simulink model "deney42"  (R2023b)
settings: Solver=VariableStepAuto  StartTime=0.0  StopTime=20  RelTol=1e-3
libraries: commrandsrc3 x1, spsControlledVoltageSourceLib x1, spsDiodeLib x1, dspfdesign x1, spsParallelRLCBranchLib x1, spsVoltageMeasurementLib x1, sps_lib x1
settings Model: Creator=fatih  LastModifiedBy=fatih

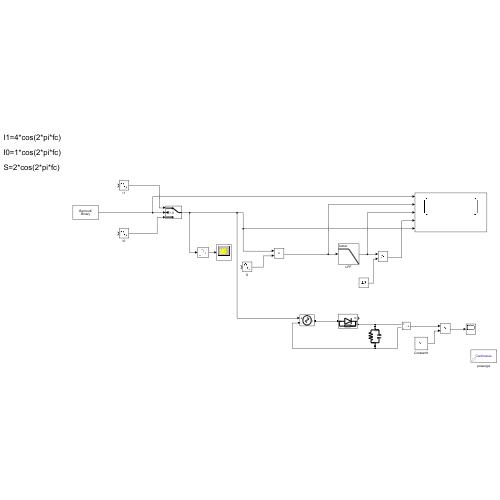
[thumbnail: Simulink's stored preview of the top-level diagram]
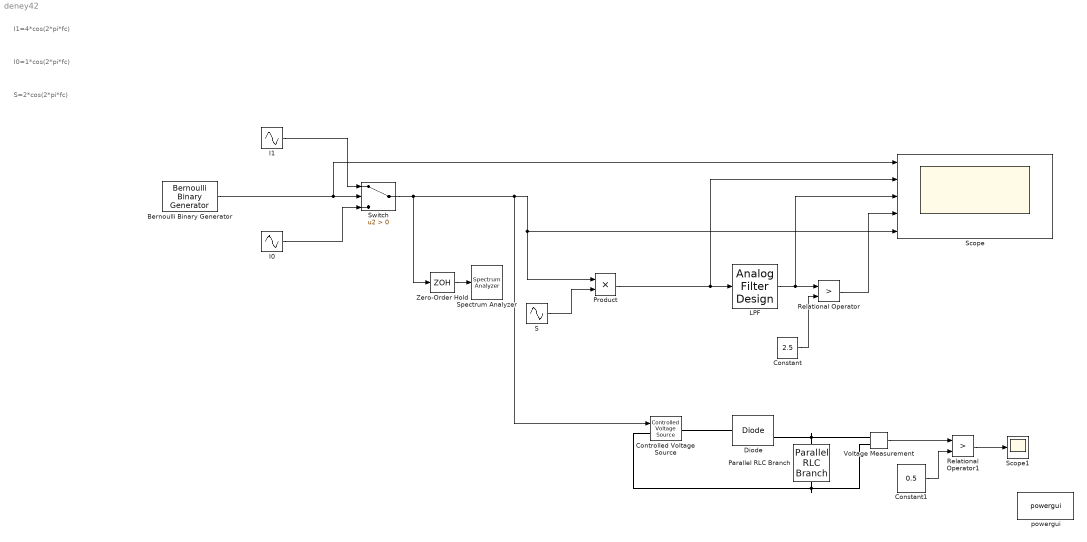
== system deney42 ==
  note: S=2*cos(2*pi*fc)
  note: I0=1*cos(2*pi*fc)
  note: I1=4*cos(2*pi*fc)
  Bernoulli Binary Generator : commrandsrc3/Bernoulli Binary Generator  ProbabilityOfZero=0.5  SeedSource=Auto  Seed=0  SampleTime=1  SamplesPerFrame=1  OutputDataType=double  SimulateUsing=Interpreted execution
  Constant : Constant  Value=2.5
  Constant1 : Constant  Value=0.5  VectorParams1D=off  SampleTime=-1
  Controlled Voltage Source : spsControlledVoltageSourceLib/Controlled Voltage Source  Initialize=on  Source_Type=AC  Amplitude=0  Phase=0  Frequency=0  Measurements=None
  Diode : spsDiodeLib/Diode  Ron=0.001  Lon=0  Vf=0.8  IC=0  UseSnubber=0  Rs=5000000  Cs=250e-9  Measurements=on
  I0 : Sin  TimeSource=Use external signal  Frequency=12.56663706  Phase=pi/2  SampleTime=0
  I1 : Sin  TimeSource=Use external signal  Amplitude=4  Frequency=12.5663706  Phase=pi/2  SampleTime=0
  LPF : dspfdesign/Analog Filter Design  method=Butterworth  filttype=Lowpass  N=8  Wlo=1.5*2*pi  Whi=80  Rp=2  Rs=40
  Parallel RLC Branch : spsParallelRLCBranchLib/Parallel RLC Branch  LConnTagsString=a  RConnTagsString=__new0  BranchType=RC  Resistance=350000  Inductance=1e-3  SetiL0=off  InitialCurrent=0  Capacitance=0.7e-6  Setx0=off  InitialVoltage=0  Measurements=None
  Product : Product
  Relational Operator : RelationalOperator  Operator=>  OutDataTypeStr=boolean  RndMeth=Simplest  InputSameDT=off
  Relational Operator1 : RelationalOperator  Operator=>  OutDataTypeStr=boolean  RndMeth=Simplest  InputSameDT=off
  S : Sin  TimeSource=Use external signal  Amplitude=2  Frequency=12.5663706  Phase=pi  SampleTime=0
  Scope : Scope  NumInputPorts=5
  Scope1 : Scope
  Spectrum Analyzer : SpectrumAnalyzer  WindowPosition=[1.000000,41.000000,1707.000000,897.000000,]  ScopeFrameLocation=window  Span=1024  StartFrequency=-512  StopFrequency=512  YLimits=[-39.27215066,47.11669635]  ShowLegend=on  ExpandToolstrip=on
      settings: OpenAtSimulationStart=off
  Switch : Switch  Criteria=u2 > Threshold  SaturateOnIntegerOverflow=off  InputSameDT=off
  Voltage Measurement : spsVoltageMeasurementLib/Voltage Measurement  PhasorSimulation=off  OutputType=Complex  PSBequivalent=0
  Zero-Order Hold : ZeroOrderHold  SampleTime=1/1024
  powergui : sps_lib/powergui  Priority=1  SimulationMode=Continuous  SampleTime=50e-6  frequency=60  Iterations=50  frequencyindice=0  Pbase=100e6  ErrMax=1e-4  UnitsV=kV  UnitsW=MW  buscounter=0  FunctionMessages=off  echomessages=off  EnableUseOfTLC=off  CurrentSourceSwitches=off  DisableSnubberDevices=off  DisableRonSwitches=off  DisableVfSwitches=off  DisplayEquations=off  AutomaticDiscreteSolvers=off  SolverType=Tustin/Backward Euler (TBE)  Interpol=off  ExternalGateDelay=off  methode=off  Ts=100  x0status=blocks  SPID=on  SwTol=0  HookPort=off  NonlinearTolerance=1e-4  nMaxIteration=100  ContinueOnMaxIteration=off  RestoreLinks=warning  ResistiveCurrentMeasurement=off  Frange=[0:2:500]  Ylog=off  Xlog=on  ShowGrid=off  save=off  variable=ZData  structure=0  ZoomFFT=off  StartTime=0.0  cycles=1  DisplayStyle=1  fundamental=60  FreqAxis=off  MaxFrequency=1000  frequencyindicesteady=1  RmsSteady=1  display=off
  wires:
  Switch/1 -> Controlled Voltage Source/1, Product/1, Scope/5, Zero-Order Hold/1
  Zero-Order Hold/1 -> Spectrum Analyzer/1
  I1/1 -> Switch/1
  I0/1 -> Switch/3
  S/1 -> Product/2
  Constant/1 -> Relational Operator/2
  Bernoulli Binary Generator/1 -> Scope/1, Switch/2
  Product/1 -> LPF/1, Scope/2
  Relational Operator/1 -> Scope/4
  LPF/1 -> Scope/3, Relational Operator/1
  Voltage Measurement/1 -> Relational Operator1/1
  Constant1/1 -> Relational Operator1/2
  Relational Operator1/1 -> Scope1/1
  connections:
  Diode/LConn1 -- Controlled Voltage Source/RConn1
  Voltage Measurement/LConn1 -- Diode/RConn1 -- Parallel RLC Branch/LConn1
  Controlled Voltage Source/LConn1 -- Parallel RLC Branch/RConn1 -- Voltage Measurement/LConn2
